simulink model "adc1_sub2_masked2"  (R2018b)
settings: Solver=ode45  StartTime=0.0  StopTime=10e-05  RelTol=1e-3  EnableMultiTasking=on
libraries: dsparch4 x2
settings Model: Creator=bbhattac  LastModifiedBy=khung
settings DataIOCC: LimitDataPoints=on  SaveFormat=Array
settings OptimizationCC: ExpressionDepthLimit=2147483647  LifeSpan=inf
settings DebuggingCC: UnderspecifiedInitializationDetection=Classic  MergeDetectMultiDrivingBlocksExec=none  SolverPrmCheckMsg=warning  ParameterPrecisionLossMsg=none  FcnCallInpInsideContextMsg=warning  StateNameClashWarn=warning  SFUnexpectedBacktrackingDiag=warning  SFNoUnconditionalDefaultTransitionDiag=warning  SFExecutionAtInitializationDiag=none
settings HardwareCC: ProdBitPerPointer=32  ProdBitPerSizeT=32  ProdBitPerPtrDiffT=32  ProdLargestAtomicFloat=None  ProdIntDivRoundTo=Undefined  ProdEndianess=Unspecified  ProdWordSize=32  ProdHWDeviceType=32-bit Generic
settings ModelReferenceCC: PropagateSignalLabelsOutOfModel=off
settings SFSimCC: SimUseLocalCustomCode=off
settings RTWCC: RTWUseLocalCustomCode=off
settings CodeAppCC: StateflowObjectComments=on
settings GRTTargetCC: TargetLangStandard=C89/C90 (ANSI)  GeneratePreprocessorConditionals=Disable all  CombineOutputUpdateFcns=off  GRTInterface=on
settings ConfigComp: CovMetricSettings=dw  CovHtmlReporting=on  CovSaveCumulativeToWorkspaceVar=on  CovSaveSingleToWorkspaceVar=on  CovExternalEMLEnable=off

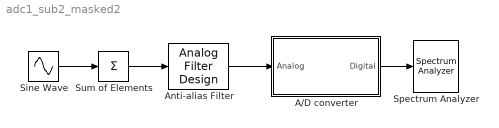
== system adc1_sub2_masked2 ==
  A/D converter : Subsystem  mask{minDelay=1.0e-9, maxDelay=5.0e-9, nonlingain=0.1, nbits=8}
      mask prompts: minDelay "Minimum aperture delay"; maxDelay "Maximum aperture delay"; nonlingain "Nonlinear gain"; nbits "No. of quantization bits"
      mask Display:
      | plot([0,1,1,2,2,3,3,4,4],[0,0,1,1,2,2,3,3,4]);
      | plot([0,4],[2,2]);
      | plot([2,2],[0,4]);
      | % Note that you don't need to specify 'hold on'
      | % to keep plotting on the same axis for the icon.
      | text(0.2,3,['ADC-',num2str(nbits)]);
  Anti-alias Filter : dsparch4/Analog Filter Design  method=Butterworth  filttype=Lowpass  N=8  Wlo=2*pi*50e+06  Whi=80  Rp=2  Rs=40
  Sine Wave : Sin  Amplitude=0.25  Frequency=2*pi*[20 22]*1e6  SampleTime=0
  Spectrum Analyzer : SpectrumAnalyzer
  Sum of Elements : Sum  Inputs=+
  wires:
  Sine Wave/1 -> Sum of Elements/1
  Sum of Elements/1 -> Anti-alias Filter/1
  Anti-alias Filter/1 -> A/D converter/1(Analog)
  A/D converter/1(Digital) -> Spectrum Analyzer/1

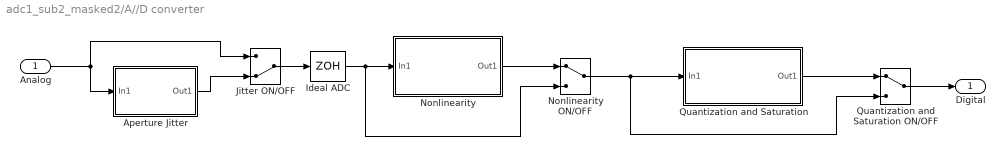
== system adc1_sub2_masked2/A//D converter ==
  Analog : Inport
  Aperture Jitter : Subsystem
  Ideal ADC : ZeroOrderHold  SampleTime=1/100e6
  Jitter ON/OFF : ManualSwitch  CurrentSetting=0
  Nonlinearity : Subsystem
  Nonlinearity ON/OFF : ManualSwitch
  Quantization and Saturation ON/OFF : ManualSwitch
  Quantization and Saturation : Subsystem
  Digital : Outport
  wires:
  Aperture Jitter/1(Out1) -> Jitter ON/OFF/2
  Quantization and Saturation ON/OFF/1 -> Digital/1
  Nonlinearity/1(Out1) -> Nonlinearity ON/OFF/1
  Nonlinearity ON/OFF/1 -> Quantization and Saturation/1(In1), Quantization and Saturation ON/OFF/2
  Quantization and Saturation/1(Out1) -> Quantization and Saturation ON/OFF/1
  Ideal ADC/1 -> Nonlinearity/1(In1), Nonlinearity ON/OFF/2
  Jitter ON/OFF/1 -> Ideal ADC/1
  Analog/1 -> Aperture Jitter/1(In1), Jitter ON/OFF/1

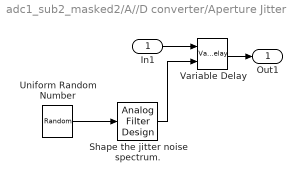
== system adc1_sub2_masked2/A//D converter/Aperture Jitter ==
  In1 : Inport
  "Shape the jitter noise spectrum. " : dsparch4/Analog Filter Design  method=Butterworth  filttype=Lowpass  N=3  Wlo=2*pi*20e6  Whi=80  Rp=2  Rs=40
  Uniform Random Number : UniformRandomNumber  Minimum=minDelay  Maximum=maxDelay  Seed=1234  SampleTime=0
  Variable Delay : VariableTransportDelay  MaximumDelay=1.1*maxDelay  ZeroDelay=on  TransDelayFeedthrough=on
  Out1 : Outport
  wires:
  Variable Delay/1 -> Out1/1
  In1/1 -> Variable Delay/1
  "Shape the jitter noise spectrum. "/1 -> Variable Delay/2
  Uniform Random Number/1 -> "Shape the jitter noise spectrum. "/1

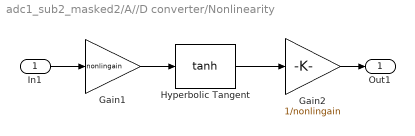
== system adc1_sub2_masked2/A//D converter/Nonlinearity ==
  In1 : Inport
  Gain1 : Gain  Gain=nonlingain  SaturateOnIntegerOverflow=on  OutDataTypeStr=Inherit: Same as input  ParamDataTypeStr=Inherit: Same as input
  Gain2 : Gain  Gain=1/nonlingain  SaturateOnIntegerOverflow=on  OutDataTypeStr=Inherit: Same as input  ParamDataTypeStr=Inherit: Same as input
  Hyperbolic Tangent : Trigonometry  Operator=tanh
  Out1 : Outport
  wires:
  Gain2/1 -> Out1/1
  In1/1 -> Gain1/1
  Gain1/1 -> Hyperbolic Tangent/1
  Hyperbolic Tangent/1 -> Gain2/1

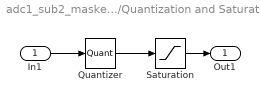
== system adc1_sub2_masked2/A//D converter/Quantization and Saturation ==
  In1 : Inport
  Quantizer : Quantizer  QuantizationInterval=2^-nbits
  Saturation : Saturate
  Out1 : Outport
  wires:
  Saturation/1 -> Out1/1
  In1/1 -> Quantizer/1
  Quantizer/1 -> Saturation/1
